simulink model "WMI"  (R2018a)
settings: Solver=ode45  StartTime=0.0  StopTime=10000  FixedStep=0.1  MaxStep=0.1  RelTol=1e-3
libraries: fuzblock x2
settings Model: Creator=hfekriaz  LastModifiedBy=hfekriaz

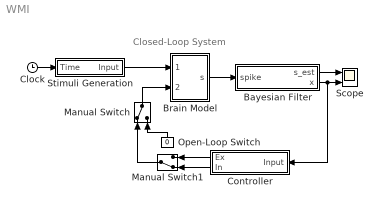
== system WMI ==
  note: Closed-Loop System
  Bayesian Filter : Subsystem
  "Brain Model " : Subsystem
  Clock : Clock
      settings: Decimation=10000
  Controller : Subsystem
  Manual Switch : ManualSwitch
  Manual Switch1 : ManualSwitch  CurrentSetting=0
  Open-Loop Switch : Constant  Value=0
  Scope : Scope  NumInputPorts=2
  "Stimuli Generation " : Subsystem
  wires:
  "Brain Model "/1("s ") -> Bayesian Filter/1(spike)
  Clock/1 -> "Stimuli Generation "/1(Time)
  "Stimuli Generation "/1("Input ") -> "Brain Model "/1(u_s)
  Bayesian Filter/1("s_est ") -> Scope/1
  Manual Switch/1 -> "Brain Model "/2(Control)
  Manual Switch1/1 -> Manual Switch/1
  Open-Loop Switch/1 -> Manual Switch/2
  Controller/1("Ex ") -> Manual Switch1/1
  Controller/2("In ") -> Manual Switch1/2
  Bayesian Filter/2(x) -> Controller/1(Input), Scope/2

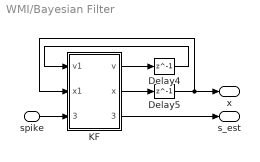
== system WMI/Bayesian Filter ==
  spike : Inport
  Delay4 : Delay  DelayLength=1  InitialCondition=0.0006
  Delay5 : Delay  DelayLength=1  InitialCondition=1.4
  KF : MATLAB Function  TreatAsAtomicUnit=on
  "s_est " : Outport
  x : Outport  Port=2
  wires:
  KF/2(x) -> Delay5/1
  KF/1(v) -> Delay4/1
  Delay4/1 -> KF/1(v1)
  Delay5/1 -> KF/2(x1), x/1
  spike/1 -> KF/3(spike)
  KF/3(s_est) -> "s_est "/1

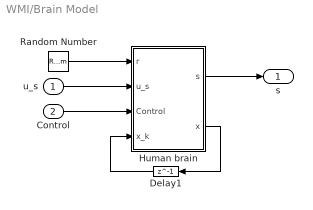
== system WMI/Brain Model  ==
  u_s : Inport
  Control : Inport  Port=2
  Delay1 : Delay  DelayLength=1  InitialCondition=1.4  InputProcessing=Inherited
  Human brain : MATLAB Function  TreatAsAtomicUnit=on
  Random Number : RandomNumber  Variance=0.00000012  Seed=55  SampleTime=1
  "s " : Outport
  wires:
  u_s/1 -> Human brain/2(u_s)
  Random Number/1 -> Human brain/1(r)
  Delay1/1 -> Human brain/4(x_k)
  Human brain/1(s) -> "s "/1
  Human brain/2(x) -> Delay1/1
  Control/1 -> Human brain/3(Control)

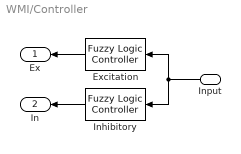
== system WMI/Controller ==
  Input : Inport
  Excitation : fuzblock/Fuzzy Logic  Controller  FIS='Ex.fis'  OutputSampleNumber=101  DataType=double  FuzzifiedInputs=off  RuleFiringStrengths=off  RuleOutputs=off  AggregatedOutputs=off  SimulateUsing=Interpreted execution  OutOfRangeInputValueMessage=warning  NoRuleFiredMessage=warning  EmptyOutputFuzzySetMessage=warning
  Inhibitory : fuzblock/Fuzzy Logic  Controller  FIS='In.fis'  OutputSampleNumber=101  DataType=double  FuzzifiedInputs=off  RuleFiringStrengths=off  RuleOutputs=off  AggregatedOutputs=off  SimulateUsing=Interpreted execution  OutOfRangeInputValueMessage=warning  NoRuleFiredMessage=warning  EmptyOutputFuzzySetMessage=warning
  "Ex " : Outport
  "In " : Outport  Port=2
  wires:
  Input/1 -> Inhibitory/1, Excitation/1
  Excitation/1 -> "Ex "/1
  Inhibitory/1 -> "In "/1

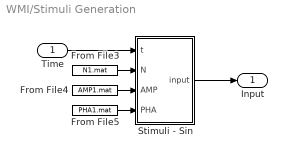
== system WMI/Stimuli Generation  ==
  Time : Inport
  From File3 : FromFile  FileName=N1.mat
  From File4 : FromFile  FileName=AMP1.mat
  From File5 : FromFile  FileName=PHA1.mat
  Stimuli - Sin : MATLAB Function  TreatAsAtomicUnit=on
  "Input " : Outport
  wires:
  Time/1 -> Stimuli - Sin/1(t)
  From File5/1 -> Stimuli - Sin/4(PHA)
  From File3/1 -> Stimuli - Sin/2(N)
  From File4/1 -> Stimuli - Sin/3(AMP)
  Stimuli - Sin/1(input) -> "Input "/1

== matlab function WMI/Bayesian Filter/KF ==
  data: v1 input; v output; x1 input; x output; spike input; s_est output
function [v,x,s_est]= fcn(v1,x1,spike)

n = spike;
M = 1;
veps = zeros(1, M + 1);
veps_guess =  0.0001;   

veps(1) = veps_guess;
mu = -2.19;
tol = 10^(-14);

v3 = v1 + veps(1);
vkj=v3;
xkj=x1;
nk=n;

it = zeros(45,1);
g= zeros(45,1);
gprime= zeros(45,1);
it(1) = xkj + vkj * (nk - exp(mu + xkj) / (1 + exp(mu + xkj)));
sol = 0;

for i = 1:40    
   g(i)     = xkj + vkj * (nk - exp(mu + it(i)) / (1 + exp(mu + it(i)))) - it(i);
   gprime(i)= (-1) * vkj * exp(mu + it(i)) / (1 + exp(mu + it(i)))^2 - 1;
   it(i+1)  = it(i) - g(i)/gprime(i);

   sol = it(i+1);
   
   if abs(sol - it(i))>tol 
      continue 
   end
end 
x = sol;
v = ((1 / (v3)) + (exp(mu + x)) / ((1 + exp(mu + x))*(1 / (1 + exp(mu + x)))))^(-1);

alpha  = -2.19;
q = 1/(1+exp(-1*(alpha +x)));
s=0;
if q>rand(1)
    s = 1;
end
s_est = s;

end

== matlab function WMI/Brain Model /Human brain ==
  settings: updateMethod=DISCRETE
  data: r input; u_s input; Control input; s output; x output; x_k input
function [s,x]  = fcn(r,u_s,Control,x_k)

x = x_k + u_s +  Control + r ;

alpha  = -2.19;
q = 1/(1+exp(-1*(alpha +x)));
s=0;
if rand(1)<q
    s = 1;
end

end

== matlab function WMI/Stimuli Generation /Stimuli - Sin ==
  data: t input; N input; AMP input; PHA input; input output
function input = fcn(t,N,AMP,PHA)
%N, AMP, PHA are comming from the offline processes to generate proper
%environemntal stimulus 

a =    -0.06484;
b =    -0.01877; 

%here our final time is T2, i.e. includes one stress and one relaxing periods

T1 = 5000; %time from first stress task to the first relaxing  period
T2 = 10000; %time from first relaxing to second stress task
T3 = 15000; %time from second stress to second relaxation period
if t < T1
    Y1 = 0;
    for i=1:length(N)
        Y1 = AMP(i)*cos(N(i)*t + PHA(i)) + Y1 ;
    end
    input = Y1;
elseif t<T2
    input  = a*exp(b*(t-T1));
elseif t<T3
    Y2 = 0;
    for i=1:length(N)
        Y2 = AMP(i)*cos(N(i)*(t - T2) + PHA(i)) + Y2;
    end
    input = Y2 + 0.0015;
else 
    input  = 1.5*a*exp(0.7*b*(t-T3));
end
input = 0.7*input;
end
